simulink model "sm_bushing_test_tr3ro3"  (R2022a)
settings: Solver=ode15s  StartTime=0.0  StopTime=12  MaxStep=1e-2  RelTol=1e-3  AbsTol=1e-3  EnableMultiTasking=on
PreLoadFcn:
  | sm_bushing_test_radial_params
undefined symbols (not defined in the file or in its folder): Visual
libraries: fl_lib x8, sm_lib x6, nesl_utility x5, linkage_bushing_6DOF_lib x1
Description:
  | Bushing Multibody Model, Radial Tests
settings Model: Creator=smiller  LastModifiedBy=smiller
settings SolverCC: AutoScaleAbsTol=off  AlgebraicLoopSolver=TrustRegion  MaxZcPerStep=1
settings DataIOCC: LimitDataPoints=on  MaxDataPoints=10000  SignalLoggingName=logsout_sm_bushing_test_tr3ro3
settings OptimizationCC: LifeSpan=inf
settings DebuggingCC: UnconnectedInputMsg=warning  UnconnectedOutputMsg=warning  UnconnectedLineMsg=warning  AllowSymbolicDim=off  SFUnexpectedBacktrackingDiag=warning  SFNoUnconditionalDefaultTransitionDiag=warning  SFExecutionAtInitializationDiag=none  SFMachineParentedDataDiag=warning  ArithmeticOperatorsInVariantConditions=warning
settings SFSimCC: SimUseLocalCustomCode=off  CustomCodeUndefinedFunction=UseInterfaceOnly
settings RTWCC: RTWUseLocalCustomCode=off  DLArmComputeVersion=19.05
settings CodeAppCC: StateflowObjectComments=on
settings GRTTargetCC: TargetLangStandard=C89/C90 (ANSI)
settings ConfigComp: CovMetricSettings=dw  CovSaveCumulativeToWorkspaceVar=on  CovSaveSingleToWorkspaceVar=on  CovExternalEMLEnable=off  CovSFcnEnable=off
settings SimscapeCC: SimscapeLogType=all  SimscapeLogSimulationStatistics=on  SimscapeLogName=simlog_sm_bushing_test_tr3ro3  SimscapeLogLimitData=off  SimscapeLogDataHistory=10000
settings ExplorerConfigSet: InternalSimMechanicsExplorerSettings="<ExplorerConfiguration><canonicalview>default</canonicalview><AnimationSetting><BasePlaybackSpeed>1.0</BasePlaybackSpeed><PlaybackSpeedFactor>4.0</PlaybackSpeedFactor></AnimationSetting><TilePanel><TileInfo><Tiles Columns=\"2\" Count=\"2\" Rows=\"1\"><Column Weight=\"0.5\"/><Column Weight=\"0.5\"/><Row Weight=\"1\"/><Tile Height=\"1\" Width=\"1\" X=\"0\" Y=\"0\"/><Tile Height=\"1\" Width=\"1\" X=\"1\" Y=\"0\"/></Tiles></TileInfo><SceneInfo><SceneViewer><BGColor><R>1</R><G>1</G><B>1</B></BGColor><Camera><DoPerspective>off</DoPerspective><Position><X>0.576528019613331555</X><Y>-0.578172549009733361</Y><Z>0.577350278311176801</Z></Position><Center><X>-0.000822249576294329038</X><Y>-0.000822279820107520718</Y><Z>9.1215509381305758e-09</Z></Center><Up><X>-0.408248290463863073</X><Y>0.408248290463863073</Y><Z>0.816496580927726145</Z></Up><ViewLimDist>1</ViewLimDist><YLim>0.435085268762739508</YLim><XLim>0.320460786521434782</XLim></Camera></SceneViewer><SceneViewer><BGColor><R>1</R><G>1</G><B>1</B></BGColor><Camera><DoPerspective>off</DoPerspective><Position><X>-0.00195245382293640635</X><Y>-0.00195245413993819228</Y><Z>1.00000004951935484</Z></Position><Center><X>-0.00195245382293640635</X><Y>-0.00195245413993819228</Y><Z>4.95193548388783711e-08</Z></Center><Up><X>0</X><Y>1</Y><Z>-0</Z></Up><ViewLimDist>1</ViewLimDist><YLim>0.307651748713474504</YLim><XLim>0.226599998772144318</XLim></Camera></SceneViewer></SceneInfo></TilePanel><MechEditorPanel><Cameras/><GfxPanelCameraMap/><VideoCreator><PlaybackSpeedRatio>1.0</PlaybackSpeedRatio><FrameRate>30</FrameRate><VideoFormat>Motion JPEG AVI</VideoFormat><FrameSize>auto</FrameSize></VideoCreator></MechEditorPanel></ExplorerConfiguration>"

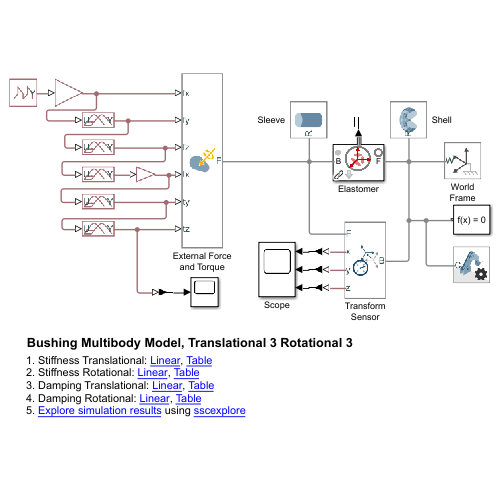
[thumbnail: Simulink's stored preview of the top-level diagram]
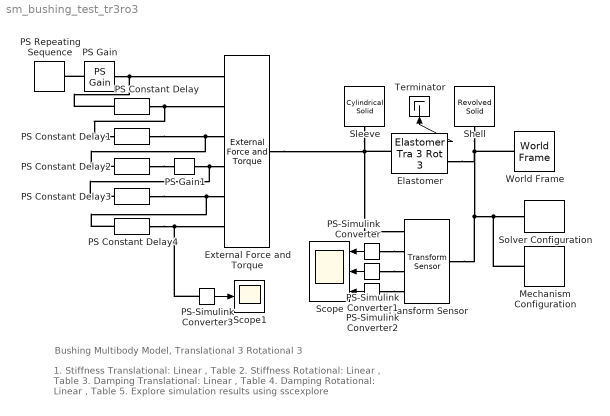
== system sm_bushing_test_tr3ro3 ==
  note: 1. Stiffness Translational: Linear , Table
      | 2. Stiffness Rotational: Linear , Table
      | 3. Damping Translational: Linear , Table
      | 4. Damping Rotational: Linear , Table
      | 5. Explore simulation results using sscexplore
  note: Bushing Multibody Model, Translational 3 Rotational 3
  Elastomer : linkage_bushing_6DOF_lib/Elastomer Tra 3 Rot 3  checkbox_setTargets=off  popup_force_law_spr_axiX=Table  k_axialX=VDatabase.Subframe_Conn.BushShock_Tr3Ro3_SLGf_MacP.SpringX.Linear.K.Value  x_axialX=VDatabase.Subframe_Conn.BushShock_Tr3Ro3_SLGf_MacP.SpringX.Table.x.Value  f_axialX_spr=VDatabase.Subframe_Conn.BushShock_Tr3Ro3_SLGf_MacP.SpringX.Table.f.Value  popup_force_law_dam_axiX=Table  d_axialX=VDatabase.Subframe_Conn.BushShock_Tr3Ro3_SLGf_MacP.DamperX.Linear.d.Value  v_axialX=VDatabase.Subframe_Conn.BushShock_Tr3Ro3_SLGf_MacP.DamperX.Table.v.Value  f_axialX_dam=VDatabase.Subframe_Conn.BushShock_Tr3Ro3_SLGf_MacP.DamperX.Table.f.Value  popup_force_law_spr_axiY=Table  k_axialY=VDatabase.Subframe_Conn.BushShock_Tr3Ro3_SLGf_MacP.SpringY.Linear.K.Value  x_axialY=VDatabase.Subframe_Conn.BushShock_Tr3Ro3_SLGf_MacP.SpringY.Table.x.Value  f_axialY_spr=VDatabase.Subframe_Conn.BushShock_Tr3Ro3_SLGf_MacP.SpringY.Table.f.Value  popup_force_law_dam_axiY=Table  d_axialY=VDatabase.Subframe_Conn.BushShock_Tr3Ro3_SLGf_MacP.DamperY.Linear.d.Value  v_axialY=VDatabase.Subframe_Conn.BushShock_Tr3Ro3_SLGf_MacP.DamperY.Table.v.Value  f_axialY_dam=VDatabase.Subframe_Conn.BushShock_Tr3Ro3_SLGf_MacP.DamperY.Table.f.Value  popup_force_law_spr_axiZ=Table  k_axialZ=VDatabase.Subframe_Conn.BushShock_Tr3Ro3_SLGf_MacP.SpringZ.Linear.K.Value  x_axialZ=VDatabase.Subframe_Conn.BushShock_Tr3Ro3_SLGf_MacP.SpringZ.Table.x.Value  f_axialZ_spr=VDatabase.Subframe_Conn.BushShock_Tr3Ro3_SLGf_MacP.SpringZ.Table.f.Value  popup_force_law_dam_axiZ=Table  d_axialZ=VDatabase.Subframe_Conn.BushShock_Tr3Ro3_SLGf_MacP.DamperZ.Linear.d.Value  v_axialZ=VDatabase.Subframe_Conn.BushShock_Tr3Ro3_SLGf_MacP.DamperZ.Table.v.Value  f_axialZ_dam=VDatabase.Subframe_Conn.BushShock_Tr3Ro3_SLGf_MacP.DamperZ.Table.f.Value  popup_force_law_spr_torX=Table  k_torsX=VDatabase.Subframe_Conn.BushShock_Tr3Ro3_SLGf_MacP.SpringqX.Linear.K.Value  q_sprX=VDatabase.Subframe_Conn.BushShock_Tr3Ro3_SLGf_MacP.SpringqX.Table.q.Value  m_sprX=VDatabase.Subframe_Conn.BushShock_Tr3Ro3_SLGf_MacP.SpringqX.Table.t.Value  popup_force_law_dam_torX=Table  d_torsX=VDatabase.Subframe_Conn.BushShock_Tr3Ro3_SLGf_MacP.DamperqX.Linear.d.Value  w_torsX=VDatabase.Subframe_Conn.BushShock_Tr3Ro3_SLGf_MacP.DamperqX.Table.w.Value  m_torsX=VDatabase.Subframe_Conn.BushShock_Tr3Ro3_SLGf_MacP.DamperqX.Table.t.Value  popup_force_law_spr_torY=Table  k_torsY=VDatabase.Subframe_Conn.BushShock_Tr3Ro3_SLGf_MacP.SpringqY.Linear.K.Value  q_sprY=VDatabase.Subframe_Conn.BushShock_Tr3Ro3_SLGf_MacP.SpringqY.Table.q.Value  m_sprY=VDatabase.Subframe_Conn.BushShock_Tr3Ro3_SLGf_MacP.SpringqY.Table.t.Value  popup_force_law_dam_torY=Table  d_torsY=VDatabase.Subframe_Conn.BushShock_Tr3Ro3_SLGf_MacP.DamperqY.Linear.d.Value  w_torsY=VDatabase.Subframe_Conn.BushShock_Tr3Ro3_SLGf_MacP.DamperqY.Table.w.Value  m_torsY=VDatabase.Subframe_Conn.BushShock_Tr3Ro3_SLGf_MacP.DamperqY.Table.t.Value  popup_force_law_spr_torZ=Table  k_torsZ=VDatabase.Subframe_Conn.BushShock_Tr3Ro3_SLGf_MacP.SpringqZ.Linear.K.Value  q_sprZ=VDatabase.Subframe_Conn.BushShock_Tr3Ro3_SLGf_MacP.SpringqZ.Table.q.Value  m_sprZ=VDatabase.Subframe_Conn.BushShock_Tr3Ro3_SLGf_MacP.SpringqZ.Table.t.Value  popup_force_law_dam_torZ=Table  d_torsZ=VDatabase.Subframe_Conn.BushShock_Tr3Ro3_SLGf_MacP.DamperqZ.Linear.d.Value  w_torsZ=VDatabase.Subframe_Conn.BushShock_Tr3Ro3_SLGf_MacP.DamperqZ.Table.w.Value  m_torsZ=VDatabase.Subframe_Conn.BushShock_Tr3Ro3_SLGf_MacP.DamperqZ.Table.t.Value  shell_or=Visual.hp.rad*2  elastomer_ir=Visual.hp.rad  shell_len=Visual.hp.rad*2  elastomer_clr=Visual.Bushing.clr  elastomer_opc=Visual.part.opc  elastomer_axis_clr=Visual.BushingXAxis.clr
  External Force and Torque : sm_lib/Forces and Torques/External Force and Torque  ForceResolutionFrame=World  EnableForceX=on  EnableForceY=on  EnableForceZ=on  EnableForce=off  TorqueResolutionFrame=World  EnableTorqueX=on  EnableTorqueY=on  EnableTorqueZ=on  EnableTorque=off
  Mechanism Configuration : sm_lib/Utilities/Mechanism Configuration  UniformGravity=Constant  GravityVector=[0 0 0]  GravityUnits=m/s^2  LinearizationDelta=0.001  JointModeTransitionNonlinearIterations=2
  PS Constant Delay : fl_lib/Physical Signals/Delays/PS Constant Delay  InputHistory=0.0 N  DelayTime=1.0 s
      settings: SourceProductBaseCode=PW,SS,VE  InternalSimscapePortConfiguration="{\"Bottom\":[],\"Left\":[{\"id\":\"U\",\"label\":\"U\",\"type\":\"input\"}],\"Right\":[{\"id\":\"Y\",\"label\":\"Y\",\"type\":\"output\"}],\"Top\":[]}"
  PS Constant Delay1 : fl_lib/Physical Signals/Delays/PS Constant Delay  InputHistory=0.0 N  DelayTime=1.0 s
      settings: SourceProductBaseCode=PW,SS,VE  InternalSimscapePortConfiguration="{\"Bottom\":[],\"Left\":[{\"id\":\"U\",\"label\":\"U\",\"type\":\"input\"}],\"Right\":[{\"id\":\"Y\",\"label\":\"Y\",\"type\":\"output\"}],\"Top\":[]}"
  PS Constant Delay2 : fl_lib/Physical Signals/Delays/PS Constant Delay  InputHistory=0.0 N  DelayTime=1.0 s
      settings: SourceProductBaseCode=PW,SS,VE  InternalSimscapePortConfiguration="{\"Bottom\":[],\"Left\":[{\"id\":\"U\",\"label\":\"U\",\"type\":\"input\"}],\"Right\":[{\"id\":\"Y\",\"label\":\"Y\",\"type\":\"output\"}],\"Top\":[]}"
  PS Constant Delay3 : fl_lib/Physical Signals/Delays/PS Constant Delay  InputHistory=0.0 N*m  DelayTime=1.0 s
      settings: SourceProductBaseCode=PW,SS,VE  InternalSimscapePortConfiguration="{\"Bottom\":[],\"Left\":[{\"id\":\"U\",\"label\":\"U\",\"type\":\"input\"}],\"Right\":[{\"id\":\"Y\",\"label\":\"Y\",\"type\":\"output\"}],\"Top\":[]}"
  PS Constant Delay4 : fl_lib/Physical Signals/Delays/PS Constant Delay  InputHistory=0.0 N*m  DelayTime=1.0 s
      settings: SourceProductBaseCode=PW,SS,VE  InternalSimscapePortConfiguration="{\"Bottom\":[],\"Left\":[{\"id\":\"U\",\"label\":\"U\",\"type\":\"input\"}],\"Right\":[{\"id\":\"Y\",\"label\":\"Y\",\"type\":\"output\"}],\"Top\":[]}"
  PS Gain : fl_lib/Physical Signals/Functions/PS Gain  gain=10000 N
      settings: SourceProductBaseCode=PW,SS,VE
  PS Gain1 : fl_lib/Physical Signals/Functions/PS Gain  gain=0.002 m
      settings: SourceProductBaseCode=PW,SS,VE
  PS Repeating Sequence : fl_lib/Physical Signals/Sources/PS Repeating Sequence  y_init=0  offset=1 s  sig_type=3  durations=[1 1 10] s  y_start=[0 1 0]  y_end=[2 10]
      settings: SourceProductBaseCode=PW,SS,VE  InternalSimscapePortConfiguration="{\"Bottom\":[],\"Left\":[],\"Right\":[{\"id\":\"Y\",\"label\":\"Y\",\"type\":\"output\"}],\"Top\":[]}"
  PS-Simulink Converter{,1..3} (4 alike) : nesl_utility/PS-Simulink Converter  PhysicalDomain=network_engine_domain  SubClassName=ps_output  LeftPortType=input  RightPortType=output  PseudoPeriodic=off  Frequencies=[]  VectorFormat=inherit  Unit=inherit  AffineConversion=off
      settings: SourceProductBaseCode=SS,PW,VE
  Scope : Scope  NumInputPorts=3
  Scope1 : Scope
  Shell : sm_lib/Body Elements/Revolved Solid  GraphicAmbientColor=[0.15 0.15 0.15 1.0]  BasedOnType=Density  CenterOfMass=[0 0 0]  CenterOfMassUnits=m  GraphicDiffuseColor=Visual.BushingShell.clr  ExportConvexHullGeometry=off  Density=1  DensityUnits=kg/m^3  DoExposeReferenceFrame=on  GraphicEmissiveColor=[0.0 0.0 0.0 1.0]  ExportEntireGeometry=off  SerializedFrames=<Frames/>  MarkerShape=Sphere  MarkerSize=10  GraphicType=FromGeometry  InertiaType=CalculateFromGeometry  Mass=1  MassUnits=kg  MomentsOfInertia=[1 1 1]  MomentsOfInertiaUnits=kg*m^2  GraphicOpacity=Visual.part.opc  ProductsOfInertia=[0 0 0]  ProductsOfInertiaUnits=kg*m^2  RevolutionCrossSection=[Visual.hp.rad*2*0.95 0.5; Visual.hp.rad*2*0.95 -0.5; Visual.hp.rad*2 -0.5; Visual.hp.rad*2 0.5].*[1 Visual.hp.rad*2]  RevolutionCrossSectionUnits=m  RevolutionAngle=180  RevolutionAngleUnits=deg  RevolutionExtent=Full  GraphicShininess=75  GraphicSpecularColor=[0.5 0.5 0.5 1.0]  GraphicVisPropType=SimpleVisualProperties
  Sleeve : sm_lib/Body Elements/Cylindrical Solid  GraphicAmbientColor=[0.15 0.15 0.15 1.0]  BasedOnType=Density  CenterOfMass=[0 0 0]  CenterOfMassUnits=m  GraphicDiffuseColor=Visual.Bushing.clr  CylinderLength=Visual.hp.rad*2  CylinderLengthUnits=m  CylinderRadius=Visual.hp.rad/2  CylinderRadiusUnits=m  Density=1  DensityUnits=kg/m^3  DoExposeReferenceFrame=on  GraphicEmissiveColor=[0.0 0.0 0.0 1.0]  ExportEntireGeometry=off  SerializedFrames=<Frames/>  MarkerShape=Sphere  MarkerSize=10  GraphicType=FromGeometry  InertiaType=CalculateFromGeometry  Mass=1  MassUnits=kg  MomentsOfInertia=[1 1 1]  MomentsOfInertiaUnits=kg*m^2  GraphicOpacity=Visual.part.opc  ProductsOfInertia=[0 0 0]  ProductsOfInertiaUnits=kg*m^2  GraphicShininess=75  GraphicSpecularColor=[0.5 0.5 0.5 1.0]  GraphicVisPropType=SimpleVisualProperties
  Solver Configuration : nesl_utility/Solver Configuration  PhysicalDomain=network_engine_domain  SubClassName=solver  LeftPortType=input  RightPortType=generic  Tones=[]  Harmonics=[]  SimulateNoise=off  Profile=off  UseLocalSampling=off  EnableSwitchedLinearOptims=on  FrequencyDomain=off  UseCCode=off  RelTol=0.001  AbsTol=1e-06  MinStep=1e-09  ToWorkspace=off  RevertToSquareIcSolve=off  NumHomotopyIterations=100  PhasorMode=off  PhasorModeNumHarmonics=1  IndexReductionMethod=DerivativeReplacement  DoDC=off  ResidualTolerance=1e-09  UseLocalSolver=off  LocalSolverChoice=NE_BACKWARD_EULER_ADVANCER  LocalSolverSampleTime=0.001  DoFixedCost=off  MaxNonlinIter=3  MaxModeIter=2  ComputeImpulses=off  ImpulseIterations=2  LinearAlgebra=Sparse  LinearAlgebraNumThread=0  EquationFormulation=NE_TIME_EF  DelaysMemoryBudget=1024  AutomaticFiltering=on  FilteringTimeConstant=0.001  PartitionStorageMethod=AS_NEEDED  PartitionMemoryBudget=1024  PartitionMethod=FAST
      settings: SourceProductBaseCode=SS,PW,VE
  Terminator : Terminator
  Transform Sensor : sm_lib/Frames and Transforms/Transform Sensor  MeasurementFrame=World  SenseAngle=off  SenseAxis=off  SenseAngle1=off  SenseAngle2=off  SenseAngle3=off  SenseQ=off  SenseR=off  SenseOmegaX=off  SenseOmegaY=off  SenseOmegaZ=off  SenseOmega1=off  SenseOmega2=off  SenseOmega3=off  SenseQDot=off  SenseRDot=off  SenseAlphaX=off  SenseAlphaY=off  SenseAlphaZ=off  SenseAlpha1=off  SenseAlpha2=off  SenseAlpha3=off  SenseQDDot=off  SenseRDDot=off  SenseX=on  SenseY=on  SenseZ=on  SenseRad=off  SenseAzim=off  SenseDist=off  SenseInc=off  SenseXDot=off  SenseYDot=off  SenseZDot=off  SenseRadDot=off  SenseAzimDot=off  SenseDistDot=off  SenseIncDot=off  SenseXDDot=off  SenseYDDot=off  SenseZDDot=off  SenseRadDDot=off  SenseAzimDDot=off  SenseDistDDot=off  SenseIncDDot=off
  World Frame : sm_lib/Frames and Transforms/World Frame
  wires:
  PS-Simulink Converter/1 -> Scope/1
  PS-Simulink Converter1/1 -> Scope/2
  Elastomer/1 -> Terminator/1
  PS-Simulink Converter2/1 -> Scope/3
  PS-Simulink Converter3/1 -> Scope1/1
  connections:
  World Frame/RConn1 -- Transform Sensor/LConn1 -- Solver Configuration/RConn1 -- Mechanism Configuration/RConn1 -- Shell/RConn1 -- Elastomer/RConn1
  Sleeve/RConn1 -- Elastomer/LConn1 -- Transform Sensor/RConn1 -- External Force and Torque/RConn1
  PS-Simulink Converter/LConn1 -- Transform Sensor/RConn2
  PS-Simulink Converter1/LConn1 -- Transform Sensor/RConn3
  PS-Simulink Converter2/LConn1 -- Transform Sensor/RConn4
  PS Gain/LConn1 -- PS Repeating Sequence/RConn1
  PS Gain/RConn1 -- PS Constant Delay/LConn1 -- External Force and Torque/LConn1
  PS Constant Delay/RConn1 -- PS Constant Delay1/LConn1 -- External Force and Torque/LConn2
  PS Constant Delay1/RConn1 -- PS Constant Delay2/LConn1 -- External Force and Torque/LConn3
  PS Constant Delay2/RConn1 -- PS Gain1/LConn1
  PS Gain1/RConn1 -- PS Constant Delay3/LConn1 -- External Force and Torque/LConn4
  PS Constant Delay3/RConn1 -- PS Constant Delay4/LConn1 -- External Force and Torque/LConn5
  PS Constant Delay4/RConn1 -- PS-Simulink Converter3/LConn1 -- External Force and Torque/LConn6
